simulink model "moving_avg_function_22b"  (R2022b)
settings: Solver=FixedStepDiscrete  StartTime=0.0  StopTime=100  RelTol=1e-3
libraries: simulink x1
settings Model: DataTypeOverride=Off  Creator=zswinnerton  LastModifiedBy=navan
settings OptimizationCC: BlockReduction=off  ConditionallyExecuteInputs=off  DefaultParameterBehavior=Inlined  InheritOutputTypeSmallerThanSingle=on
settings DebuggingCC: AlgebraicLoopMsg=error  SingleTaskRateTransMsg=error
settings HardwareCC: ProdBitPerPointer=32  ProdBitPerSizeT=32  ProdBitPerPtrDiffT=32  ProdLargestAtomicFloat=None  ProdIntDivRoundTo=Undefined  ProdEndianess=Unspecified  ProdWordSize=32  ProdHWDeviceType=ASIC/FPGA->ASIC/FPGA  TargetBitPerPointer=64  TargetBitPerSizeT=64  TargetBitPerPtrDiffT=64  TargetLongLongMode=on  TargetIntDivRoundTo=Zero  TargetEndianess=LittleEndian  TargetWordSize=64  TargetHWDeviceType=Custom Processor->MATLAB Host Computer  ProdEqTarget=off

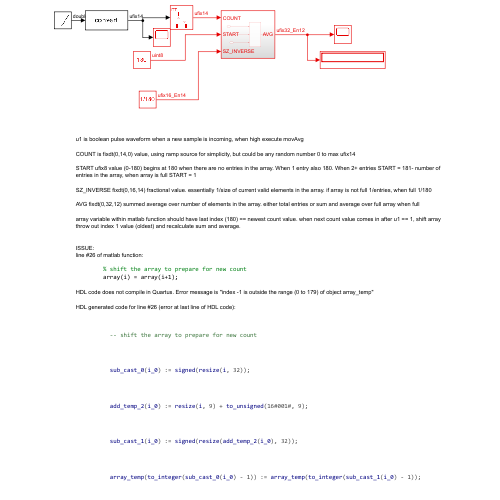
[thumbnail: Simulink's stored preview of the top-level diagram]
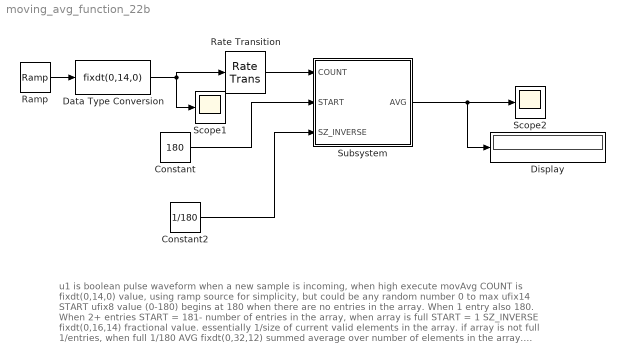
== system moving_avg_function_22b ==
  note: u1 is boolean pulse waveform when a new sample is incoming, when high execute movAvg
      |
      | COUNT is fixdt(0,14,0) value, using ramp source for simplicity, but could be any random number 0 to max ufix14
      |
      | START ufix8 value (0-180) begins at 180 when there are no entries in the array. When 1 entry also 180. When 2+ entries START = 181- number of entries in the array, when array is full START = 1
      |
      | SZ_INVERSE fixdt(0,16,14) fractional value. essentially 1/size of current valid elements in the array. if array is not full 1/entries, when full 1/180
      |
      | AVG fixdt(0,32,12) summed average over number of elements in the array. either total entries or sum and average over full array when full
      |
      | array variable within matlab function should have last index (180) == newest count value. when next count value comes in after u1 == 1, shift array throw out index 1 value (oldest) and recalculate sum and average.
      |
      | ISSUE:
      | line #26 of matlab function:
      |
      | % shift the array to prepare for new count
      | array(i) = array(i+1);
      |
      | HDL code does not compile in Quartus. Error message is "index -1 is outside the range (0 to 179) of object array_temp"
      |
      | HDL generated code for line #26 (error at last line of HDL code):
      | - - shift the array to prepare for new count
      |
      | s ub_cast_0 ( i _0 ) : = s igned ( r esize ( i , 3 2 ) ) ;
      |
      | a dd_temp_2 ( i _0 ) : = r esize ( i , 9 ) + t o_unsigned ( 1 6 # 0 01 # , 9 ) ;
      |
      | s ub_cast_1 ( i _0 ) : = s igned ( r esize ( a dd_temp_2 ( i _0 ) , 3 2 ) ) ;
      |
      | a rray_temp ( t o_integer ( s ub_cast_0 ( i _0 ) - 1 ) ) : = a rray_temp ( t o_integer ( s ub_cast_1 ( i _0 ) - 1 ) ) ;
  Constant : Constant  Value=180  OutDataTypeStr=fixdt(0,8,0)  SampleTime=0.01
  Constant2 : Constant  Value=1/180  OutDataTypeStr=fixdt(0,16,14)  SampleTime=0.01
  Data Type Conversion : DataTypeConversion  OutDataTypeStr=fixdt(0,14,0)  SaturateOnIntegerOverflow=off  RndMeth=Floor
  Display : Display
  Ramp : simulink/Sources/Ramp  slope=300  start=0  InitialOutput=0
  Rate Transition : RateTransition  OutPortSampleTime=0.01
  Scope1 : Scope
  Scope2 : Scope
  Subsystem : Subsystem
  wires:
  Data Type Conversion/1 -> Rate Transition/1, Scope1/1
  Ramp/1 -> Data Type Conversion/1
  Subsystem/1(AVG) -> Display/1, Scope2/1
  Constant/1 -> Subsystem/2(START)
  Constant2/1 -> Subsystem/3(SZ_INVERSE)
  Rate Transition/1 -> Subsystem/1(COUNT)

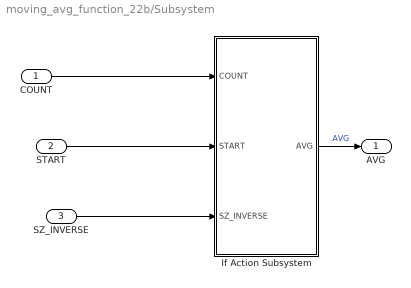
== system moving_avg_function_22b/Subsystem ==
  COUNT : Inport
  START : Inport  Port=2
  SZ_INVERSE : Inport  Port=3
  If Action Subsystem : Subsystem  TreatAsAtomicUnit=on
  AVG : Outport
  wires:
  START/1 -> If Action Subsystem/2(START)
  If Action Subsystem/1(AVG) -> AVG/1  "AVG"
  COUNT/1 -> If Action Subsystem/1(COUNT)
  SZ_INVERSE/1 -> If Action Subsystem/3(SZ_INVERSE)

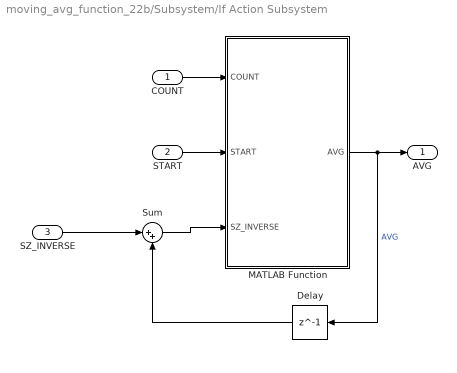
== system moving_avg_function_22b/Subsystem/If Action Subsystem ==
  COUNT : Inport
  START : Inport  Port=2
  SZ_INVERSE : Inport  Port=3
  Delay : Delay  DelayLength=1
  MATLAB Function : MATLAB Function  TreatAsAtomicUnit=on
  Sum : Sum  Inputs=|++  OutDataTypeStr=fixdt(0,16,14)
  AVG : Outport  InitialOutput=0
  wires:
  COUNT/1 -> MATLAB Function/1(COUNT)
  START/1 -> MATLAB Function/2(START)
  MATLAB Function/1(AVG) -> AVG/1, Delay/1  "AVG"
  Sum/1 -> MATLAB Function/3(SZ_INVERSE)
  SZ_INVERSE/1 -> Sum/1
  Delay/1 -> Sum/2

== matlab function moving_avg_function_22b/Subsystem/If Action Subsystem/MATLAB Function ==
  data: COUNT input fixdt(0,14,0) size=1; AVG output fixdt(0,32,12) size=1; START input fixdt(0,8,0) size=1; SZ_INVERSE input fixdt(0,16,14) size=1
function AVG = movAvg(COUNT, START, SZ_INVERSE)
%error is on line 182 of HDL code
%index -1 is outside of the range (0 to 179) of object array_temp

% Example: [ 1 2 3 4 5 6 7 8 9 10 ]
% start with 1 new entry at index 10, so only sum and average over index 10
% 2+ entries, start = (11-entries) and sum/avg all elements up to index 10
% once array is full start = 1
% This is to avoid initial array of all 0s pulling average down on startup


%#codegen
persistent array prev_count
if isempty(array)
    array = fi(zeros(1,180),0,14,0);
    prev_count = fi(zeros(1,1),0,14,0);
end

sum = fi(0,0,32,7);
% if start < 180, sum internal elements of array, otherwise just sum last element
% if START < fi(180,0,8,0)
    % lower_limit to index 179
    % for i = START:179
    for i = cast(1,'like',START):179
        
        if i >= START && START < fi(180,0,8,0)
            if i == 179
                array(180) = prev_count;
            end

            idx = i + 1;
            sum = fi(sum + array(idx),0,32,7);

            % shift the array to prepare for new count
            array(i) = array(idx);
        end
    end
% end


% add new count value to array at the end (index 180)
% array(180) = COUNT;
prev_count = COUNT;
% add last element (new count) to sum
% sum = fi(sum + array(180),0,32,7);
sum = fi(sum + prev_count,0,32,7);

AVG = fi(sum * SZ_INVERSE,0,32,12);
end
